simulink model "Overtaking_master"  (R2024a)
settings: Solver=VariableStepAuto  StartTime=0.0  StopTime=10.0  RelTol=1e-3
undefined symbols (not defined in the file): route1_frenet, route1_waypoint, route2_frenet, route2_waypoint, route3_frenet, route3_waypoint, route4_frenet, route4_waypoint, route5_frenet, route5_waypoint
libraries: CarMaker4SL x48
(part 2 of 2)

== matlab function Overtaking_master/Waypoint_Follower1 ==
  settings: sampleTime=0.1
  data: local_waypoints input; steering_angle output; state input; change_dist input; target_idx output
% local tracking
function [steering_angle, target_idx] = waypoint_follower(local_waypoints, state, change_dist)

    WHEEL_BASE = 2.9;
    lookahead_dist = 6.0;
    
    % % sigmoid lookahead_dist change
    % if(change_dist > 1.8) 
    %     lookahead_dist = (10 / (1 + exp(-0.4 * change_dist))) + 5;
    % end
    % 
    % % final state -> parking area entry
    % if(state == 7)
    %     lookahead_dist = 2.5;
    % end

    target_idx = -1;
    final_ld = 0;

    for i = 1:size(local_waypoints, 1)
        dist = norm(local_waypoints(i, :));
        if dist > lookahead_dist && local_waypoints(i, 1) > 0
            target_idx = i;
            final_ld = dist;
            break;
        end
    end

    if target_idx == -1
        steering_angle = 0;
        return;
    end

    target_point = local_waypoints(target_idx, :);
    alpha = atan2(target_point(2), target_point(1));
    alpha = wrapToPi(alpha);

    final_ld = min(max(final_ld, 2.0), 20.0); 

    steering_angle = atan2(2 * WHEEL_BASE * sin(alpha), final_ld);
end


% % global tracking
% function [steering_angle, start_idx] = pure_pursuit(waypoints, vehicle_position, head)
% 
%     persistent last_target_idx;
%     if isempty(last_target_idx)
%         last_target_idx = 1; % 초기값 설정
%     end
% 
%     WHEEL_BASE = 2.7;
% 
%     waypoints_x = waypoints(:,1);
%     waypoints_y = waypoints(:,2);
%     % num_points = length(waypoints_x);
%     num_points = 300;
% 
%     local_waypoints = zeros(num_points, 2);
%     x_ego = vehicle_position(1);
%     y_ego = vehicle_position(2);
% 
%     for i = 1:num_points
%         dx = waypoints_x(i) - x_ego;
%         dy = waypoints_y(i) - y_ego;
% 
%         local_x = dx * cos(-head) - dy * sin(-head);
%         local_y = dx * sin(-head) + dy * cos(-head);
% 
%         local_waypoints(i, :) = [local_x, local_y];
%     end    
% 
%     lookahead_dist = 5.0;
% 
%     distances_to_waypoints = sqrt((waypoints_x - x_ego).^2 + (waypoints_y - y_ego).^2);
%     [~, closest_idx] = min(distances_to_waypoints);
% 
%     start_idx = max(last_target_idx, closest_idx);
% 
%     target_idx = -1;
%     final_ld = 0;
%     for i = start_idx:num_points
%         dist = norm(local_waypoints(i, :));
%         if dist > lookahead_dist && local_waypoints(i, 1) > 0
%             target_idx = i;
%             final_ld = dist;
%             break;
%         end
%     end
% 
%     if target_idx == -1
%         for i = 1:start_idx-1
%             dist = norm(local_waypoints(i, :));
%             if dist > lookahead_dist && local_waypoints(i, 1) > 0
%                 target_idx = i;
%                 final_ld = dist;
%                 break;
%             end
%         end
%     end
% 
%     if target_idx == -1
%         steering_angle = 0;
%         return;
%     end
% 
%     target_point = local_waypoints(target_idx, :);
%     alpha = atan2(target_point(2), target_point(1));
%     alpha = wrapToPi(alpha);
% 
%     final_ld = min(max(final_ld, 2.0), 20.0);
% 
%     steering_angle = atan2(2 * WHEEL_BASE * sin(alpha), final_ld);
% 
%     last_target_idx = target_idx;
% end

== matlab function Overtaking_master/MATLAB Function1 ==
  data: lane_id input; route_waypoint output; route_frenet output; route1_waypoint input; route1_frenet input; route2_waypoint input; route2_frenet input; route3_waypoint input; route3_frenet input; route4_waypoint input; route4_frenet input; route5_waypoint input; route5_frenet input
function [route_waypoint, route_frenet] = select_lane(lane_id, route1_waypoint, ...
    route1_frenet, route2_waypoint, route2_frenet, route3_waypoint, route3_frenet, ...
    route4_waypoint, route4_frenet, route5_waypoint, route5_frenet)

    [route_waypoint, route_frenet] = select_lane_func(lane_id, route1_waypoint, ...
    route1_frenet, route2_waypoint, route2_frenet, route3_waypoint, route3_frenet, ...
    route4_waypoint, route4_frenet, route5_waypoint, route5_frenet);
end
